simulink model "Falcon"  (R2025b)
settings: Solver=ode1  StartTime=0.0  StopTime=inf  FixedStep=Controller_Sample_Time  RelTol=1e-3  EnableMultiTasking=on
values from neighbouring files (symbols this model uses):
  angles_qcar2 = angles_new_qcar2(2: length (angles_new_qcar2), width (angles_new_qcar2)-5)    [Setup_QCar2_Params.m]
  cal_pos = [0, 0, 0]    [Setup_QCar2_Params.m]
  Controller_Sample_Time = 1/500    (= 0.002)    [Setup_QCar2_Params.m]
  CSI_Sample_Time = Controller_Sample_Time * ceil(0.033 / Controller_Sample_Time)    [Setup_QCar2_Params.m]
  GyroKF_P0 = eye(2)    [Setup_QCar2_Params.m]
  GyroKF_Q = diag([0.01, 0.001])    [Setup_QCar2_Params.m]
  GyroKF_R = 0.01    [Setup_QCar2_Params.m]
  GyroKF_X0 = [0;0]    [Setup_QCar2_Params.m]
  ImageDisplay_Sample_Time = Controller_Sample_Time * 50    (= 0.1)    [Setup_QCar2_Params.m]
  Initialization_Time = 5    [Setup_QCar2_Params.m]
  LiDAR_Sample_Time = Controller_Sample_Time * ceil(1/15 / Controller_Sample_Time)    [Setup_QCar2_Params.m]
  path_x4 = path_x2    [Setup_QCar2_Params.m]
  path_y4 = path_y2    [Setup_QCar2_Params.m]
  qcar2_lidar_to_body_rotation = -pi    (= -3.14159265359)    [Setup_QCar2_Params.m]
  qcar2_lidar_to_map_rotation = 2*pi/180    (= 0.0349065850399)    [Setup_QCar2_Params.m]
  qcar2_virtual_to_physical_lidar_rotation = 0    [Setup_QCar2_Params.m]
  QCarEKF_L = 0.256    [Setup_QCar2_Params.m]
  QCarEKF_P0 = eye(3)    [Setup_QCar2_Params.m]
  QCarEKF_Q = diag([0.00001, 0.00001, 0.00001])    [Setup_QCar2_Params.m]
  QCarEKF_R_combined = diag([0.1, 0.1, 0.01])    [Setup_QCar2_Params.m]
  QCarEKF_R_heading = diag(0.1)    [Setup_QCar2_Params.m]
  QcarKF_X0 = [0; 0; 0]    [Setup_QCar2_Params.m]
  range_qcar2 = distance_new_qcar2(2: length (distance_new_qcar2), width (distance_new_qcar2)-5)    [Setup_QCar2_Params.m]
  RealSense_Sample_Time = Controller_Sample_Time * ceil(0.033 / Controller_Sample_Time)    [Setup_QCar2_Params.m]
  steering_Kd = 0.1    [Setup_QCar2_Params.m]
  steering_Kp = 1    [Setup_QCar2_Params.m]
undefined symbols (not defined in the file or in its folder): AAAF5050, gcbh, height, HIL, JPEG, K12, left, MC, Point, qc_get_step_size, top, video_display_show, width
libraries: quarc_library x45, simulink x3, simulink_extras x3, visionanalysis x1, visiontextngfix x1
(part 3 of 3)

== matlab function Falcon/stateEstimation/Gyro KF + EKF/Heading Kalman Filter ==
  settings: updateMethod=DISCRETE
  data: thd_gyro input; th_gps input; newGPSData input; GyroKF_Q parameter; GyroKF_R parameter; GyroKF_X0 parameter; GyroKF_P0 parameter; th_hat output; gyro_bias output; Controller_Sample_Time parameter
function [th_hat, gyro_bias] = GyroKF(thd_gyro, th_gps, newGPSData, GyroKF_Q, GyroKF_R, GyroKF_X0, GyroKF_P0, Controller_Sample_Time)

    persistent X_hat P I A B C
    if isempty(X_hat)
        % State and Covarience estimates
        X_hat = GyroKF_X0;
        P = GyroKF_P0;

        % Statespace model matrices
        I = eye(2);
        A = I + Controller_Sample_Time*[0, -1;
                                   0, 0];
        B = Controller_Sample_Time*[1;
                               0];
        C = [1, 0];
    end

    % Prediction
    X_hat = A*X_hat + B*thd_gyro;
    P = A*P*A' + GyroKF_Q;

    % Correction 
    if newGPSData
        P_times_CTransposed = P*C';
        S = C*P_times_CTransposed + GyroKF_R;
        K = P_times_CTransposed / S;

        z = wrapToPi(th_gps - C*X_hat);

        X_hat = X_hat + K*z;
        X_hat(1) = wrapToPi(X_hat(1));

        P = (I - K*C) * P;
    end
    
    th_hat = X_hat(1);
    gyro_bias = X_hat(2);
end

== matlab function Falcon/stateEstimation/Gyro KF + EKF/QCar EKF ==
  settings: updateMethod=DISCRETE
  data: speed input; delta input; x_gps input; Xhat output; y_gps input; th_hat input; newGPSData input; Controller_Sample_Time parameter; QCarEKF_P0 parameter; QcarKF_X0 parameter; QCarEKF_R_heading parameter; QCarEKF_Q parameter; QCarEKF_L parameter; QCarEKF_R_combined parameter
function Xhat  = QCarEKF(speed, delta, x_gps, y_gps, th_hat, newGPSData, Controller_Sample_Time, QCarEKF_P0, QcarKF_X0, QCarEKF_R_heading, QCarEKF_Q, QCarEKF_L, QCarEKF_R_combined)




    persistent X_hat P I C_heading C_combined
    if isempty(X_hat)
        % State and Covarience estimates
        X_hat = QcarKF_X0;
        P = QCarEKF_P0;

        % Statespace model matrices
        I = eye(3);
        
        C_heading = [0, 0, 1];
        C_combined = eye(3);
    end
    
    dt = Controller_Sample_Time;
    x = X_hat(1);
    y = X_hat(2);
    th = X_hat(3);
    
    % Prediction:
    F = [1, 0, -dt*speed*sin(th);
         0, 1,  dt*speed*cos(th);
         0, 0,             1];
    P = F*P*F' + QCarEKF_Q;
    
    X_hat = X_hat + dt*speed * [cos(th);
                            sin(th);
                            tan(delta) / QCarEKF_L];
                         
    
    % Correction
    if newGPSData
        y = [x_gps; y_gps; th_hat];
        C = C_combined;
        R = QCarEKF_R_combined;
        
    else
        y = th_hat;
        C = C_heading;
        R = QCarEKF_R_heading;
    end

    P_times_CTransposed = P*C';
    S = C*P_times_CTransposed + R;
    K = P_times_CTransposed / S;

    z = y - C*X_hat;
    if newGPSData
        z(3) = wrapToPi(z(3));
    else
        z = wrapToPi(z);
    end

    X_hat = X_hat + K*z;
    X_hat(3) = wrapToPi(X_hat(3));

    P = (I - K*C) * P;
    
    Xhat = X_hat;
end

== matlab function Falcon/lidarLocalization/Match Scans/MATLAB Function ==
  data: new_range output size=SPR_qcar2 [..SPR_qcar2]; range input [1..SPR_qcar2]; angles input [1..SPR_qcar2]; new_angles output size=SPR_qcar2 [..SPR_qcar2]
function [new_range, new_angles]  = clean_zero_readings(range, angles)
range_indicies = find (range == 0);
range(range_indicies) = [];
angles(range_indicies) = [];
new_range = range;
new_angles = angles;
end

== matlab function Falcon/pathPlanner/Path 4  Look Ahead Generator/Windowed Closest Point Locator *Feedback the location1 ==
  data: x input; location output; y input; x_array input; y_array input; window input; global_search input; distance output; previous_location input
function [location,distance] = find_closest_window_point(x,y,x_array,y_array, window, global_search, previous_location)
distance = 1e6;
location = previous_location;
array_length = length (x_array);

if (global_search == 1)
    
    %Search the whole array (usually at startup)
    for i =1:array_length
        d = (x-x_array(i))^2 + (y-y_array(i))^2;
        if d < distance
            distance = d;
            location = i;
        end
    end
    
else
    
    if (location + window) > array_length
        %We need to wrap from the end
        % loop one - end of array:
        for i = (location-window):array_length
            d = (x-x_array(i))^2 + (y-y_array(i))^2;
            if d < distance
                distance = d;
                location = i;
            end
        end
        % loop two - start of array:
        for i = 1:(location+window-array_length)
            d = (x-x_array(i))^2 + (y-y_array(i))^2;
            if d < distance
                distance = d;
                location = i;
            end
        end
        
    elseif (location-window) < 1
        %We need to wrap from the beginning
        % loop one - end of array:
        for i = (array_length+location-window):array_length
            d = (x-x_array(i))^2 + (y-y_array(i))^2;
            if d < distance
                distance = d;
                location = i;
            end
        end
        % loop two - start of array:
        for i = 1:(location+window)
            d = (x-x_array(i))^2 + (y-y_array(i))^2;
            if d < distance
                distance = d;
                location = i;
            end
        end
        
    else
        %no need to wrap
        for i = (location-window):(location+window)
            d = (x-x_array(i))^2 + (y-y_array(i))^2;
            if d < distance
                distance = d;
                location = i;
            end
        end
    end
    
end
distance = sqrt(distance);
end

== matlab function Falcon/MATLAB Function ==
  data: bboxes input; distance_to_object output; labels input; scores input; depthImg input; object_class output
function [distance_to_object, object_class] = getObjectDepthClass(bboxes, labels, scores, depthImg)

% Default outputs
distance_to_object = single(-1);   % no valid detection / no valid depth
object_class = labels(1);          % placeholder only; ignore when distance_to_object < 0

bestIdx = 0;
bestScore = single(0);

% Pick the detection with the highest positive confidence
for i = 1:size(bboxes,1)
    if isfinite(scores(i)) && ...
       (scores(i) > bestScore) && ...
       (bboxes(i,3) > 1) && ...
       (bboxes(i,4) > 1)

        bestScore = scores(i);
        bestIdx = i;
    end
end

% Only continue if a real detection exists
if bestIdx > 0
    % Return detected class
    object_class = labels(bestIdx);

    % Bounding box = [x y w h]
    x = double(bboxes(bestIdx,1));
    y = double(bboxes(bestIdx,2));
    w = double(bboxes(bestIdx,3));
    h = double(bboxes(bestIdx,4));

    % Depth image size
    H = size(depthImg,1);
    W = size(depthImg,2);

    % Use a small patch around the bbox center
    cx = round(x + w/2);
    cy = round(y + h/2);

    halfW = max(1, round(0.1*w));
    halfH = max(1, round(0.1*h));

    x1 = max(1, cx - halfW);
    x2 = min(W, cx + halfW);
    y1 = max(1, cy - halfH);
    y2 = min(H, cy + halfH);

    % Average valid depth values in the center patch
    sumDepth = single(0);
    count = 0;

    for r = y1:y2
        for c = x1:x2
            d = single(depthImg(r,c));
            if isfinite(d) && (d > 0)
                sumDepth = sumDepth + d;
                count = count + 1;
            end
        end
    end

    % If depth is valid, output it
    if count > 0
        distance_to_object = sumDepth / single(count);

        % Uncomment only if RealSense depth is in millimeters
        % distance_to_object = distance_to_object / 1000;
    else
        % Detection exists but no valid depth in the selected patch
        distance_to_object = single(-1);
    end
end

== matlab function Falcon/PathPlanner ==
  settings: updateMethod=DISCRETE
  data: currentPATHXY input; measuredSpeed input; reset input; Ts input; pickupNode input; dropoffNode input; distance_to_object input; object_class input; targetSpeed output; rgbPct output; leds16 output; rideState output
function [targetSpeed, rgbPct, leds16, rideState] = Main_FSM( ...
    currentPATHXY, measuredSpeed, reset, Ts, pickupNode, dropoffNode, ...
    distance_to_object, object_class)
% =========================================================================
% Perception-Integrated Ride Logic:
%   1) If distance_to_object == -1 -> no perception override
%   2) If distance_to_object <= 1.0 m and STOP SIGN detected:
%         stop for 3.0 s, then continue
%   3) If 1.0 m < distance_to_object <= 1.7 m and RED LIGHT detected:
%         stop and wait until red light disappears
%   4) If GREEN LIGHT detected:
%         no change
%
% NOTE:
%   object_class is assumed to be a numeric/enum class ID.
%   Replace STOP_LABEL_ID, RED_LIGHT_LABEL_ID, GREEN_LIGHT_LABEL_ID below
%   with your actual detector label IDs.
% =========================================================================

% -------------------------
% Detector label IDs (EDIT THESE)
% -------------------------
STOP_LABEL_ID        = int32(3);
RED_LIGHT_LABEL_ID   = int32(2);
GREEN_LIGHT_LABEL_ID = int32(1);

% -------------------------
% Node list (ID -> [x,y])  (26 nodes: 0..25)
% -------------------------
NODE_XY = [ ...
     0.0    ,  0.0   ;  % 0
     0.269  , -0.049 ;  % 1
     1.127  , -1.075 ;  % 2
     1.127  , -0.820 ;  % 3
     2.255  , -0.049 ;  % 4
     1.984  , -0.049 ;  % 5
     1.013  ,  1.081 ;  % 6
     1.235  ,  0.791 ;  % 7
    -0.749  ,  1.077 ;  % 8
    -0.749  ,  0.790 ;  % 9
    -1.282  , -0.59  ;  % 10 (HUB)
     0.0    ,  2.033 ;  % 11
     0.0    ,  1.72  ;  % 12
     0.269  ,  1.72  ;  % 13
     2.255  ,  2.837 ;  % 14
     1.984  ,  1.72  ;  % 15
     0.908  ,  3.58  ;  % 16
     1.466  ,  3.02  ;  % 17
     0.623  ,  2.937 ;  % 18
     0.792  ,  2.729 ;  % 19
     0.0    ,  4.421 ;  % 20
     0.0    ,  4.146 ;  % 21
    -1.984  ,  2.837 ;  % 22
    -1.716  ,  2.837 ;  % 23
    -0.826  ,  3.645 ;  % 24
    -0.857  ,  1.716 ]; % 25

% -------------------------
% Clamp node IDs to valid range [0..25]
% -------------------------
pn = int32(pickupNode);
dn = int32(dropoffNode);
if pn < 0,  pn = int32(0);  end
if pn > 25, pn = int32(25); end
if dn < 0,  dn = int32(0);  end
if dn > 25, dn = int32(25); end

% -------------------------
% Points (meters)
% -------------------------
P0 = NODE_XY(10+1, :).';
P1 = NODE_XY(pn+1,  :).';
P8 = NODE_XY(dn+1,  :).';

% -------------------------
% Parameters
% -------------------------
V_DES_NORMAL      = 0.40;
V_DES_STARTUP     = 0.04;
V_DES_STOPPING    = 0.0;
STARTUP_TIME      = 6.0;

ARRIVE_RADIUS_PICKUP  = 0.30;
ARRIVE_RADIUS_DROPOFF = 0.30;
ARRIVE_RADIUS_HUB     = 0.45;

STOP_SPEED_TH      = 0.05;
STOP_HOLD_TIME     = 3.0;   % standard node stop time
STOP_SIGN_HOLD_SEC = 3.0;   % stop sign hold time

% -------------------------
% Perception distance thresholds
% -------------------------
STOP_SIGN_DIST_MAX = 1;
RED_LIGHT_DIST_MIN = 1;
RED_LIGHT_DIST_MAX = 3;

% -------------------------
% Colors (0..1)
% -------------------------
MAGENTA = [1; 0; 1];
GREEN   = [0; 1; 0];
BLUE    = [0; 0; 1];
ORANGE  = [1; 0.6; 0];
RED     = [1; 0; 0];

% -------------------------
% Car lights
% -------------------------
leds16 = false(16,1);
BRAKES = [11 12 13 14];

% -------------------------
% State machine + timers
% -------------------------
persistent s stopT time arrived1 arrived8 arrived0 spDone lastPick lastDrop
persistent stopSignTimer stopSignActive stopSignServed

if isempty(s) || reset
    s = uint8(0);
    stopT = 0;
    time  = 0;

    stopSignTimer  = 0;
    stopSignActive = false;
    stopSignServed = false;

    arrived1 = false;
    arrived8 = false;
    arrived0 = false;
    spDone = false;
    lastPick = pn;
    lastDrop = dn;
else
    if (pn ~= lastPick) || (dn ~= lastDrop)
        s = uint8(0);
        stopT = 0;
        time  = 0;

        stopSignTimer  = 0;
        stopSignActive = false;
        stopSignServed = false;

        arrived1 = false;
        arrived8 = false;
        arrived0 = false;
        spDone = false;
        lastPick = pn;
        lastDrop = dn;
    end
end

time = time + Ts;

if time < STARTUP_TIME
    V_DES = V_DES_STARTUP;
else
    V_DES = V_DES_NORMAL;
end

% -------------------------
% Current path XY + optional stop flag
% -------------------------
x = currentPATHXY(1);
y = currentPATHXY(2);

stopPoint = false;
if numel(currentPATHXY) >= 3
    stopPoint = (currentPATHXY(3) > 0.5);
end

if ~stopPoint
    spDone = false;
end

d0 = hypot(x - P0(1), y - P0(2));
d1 = hypot(x - P1(1), y - P1(2));
d8 = hypot(x - P8(1), y - P8(2));

% -------------------------
% Stop timer logic
% -------------------------
isStopped = abs(measuredSpeed) < STOP_SPEED_TH;
if isStopped
    stopT = stopT + Ts;
else
    stopT = 0;
end
fullStop = (stopT >= STOP_HOLD_TIME);

% -------------------------
% Drive-state check
% -------------------------
isDriveState = (s==uint8(1)) || (s==uint8(3)) || (s==uint8(5));

% -------------------------
% Perception logic from distance + object class
% -------------------------
validObject = isfinite(distance_to_object) && (distance_to_object >= 0);
objCode = int32(object_class);

isStopSign = validObject && ...
             (distance_to_object <= STOP_SIGN_DIST_MAX) && ...
             (objCode == STOP_LABEL_ID);

isRedLight = validObject && ...
             (distance_to_object > RED_LIGHT_DIST_MIN) && ...
             (distance_to_object <= RED_LIGHT_DIST_MAX) && ...
             (objCode == RED_LIGHT_LABEL_ID);

isGreenLight = validObject && ...
               (objCode == GREEN_LIGHT_LABEL_ID); %#ok<NASGU>

% Re-arm stop sign only after it disappears
if ~isStopSign && ~stopSignActive
    stopSignServed = false;
end

% -------------------------
% Stop-sign override
% Stop 3 seconds, then continue
% Only in drive states
% -------------------------
if isDriveState && isStopSign && ~stopSignActive && ~stopSignServed
    stopSignActive = true;
    stopSignTimer = 0;
end

if stopSignActive
    targetSpeed = V_DES_STOPPING;
    rgbPct = RED;
    leds16(BRAKES) = true;

    stopSignTimer = stopSignTimer + Ts;

    if stopSignTimer >= STOP_SIGN_HOLD_SEC
        stopSignActive = false;
        stopSignServed = true;
        stopSignTimer = 0;
        stopT = 0;
    end

    rideState = double(s);
    return;
end

% -------------------------
% Red-light override
% Stop until red light disappears
% Only in drive states
% -------------------------
if isDriveState && isRedLight
    targetSpeed = V_DES_STOPPING;
    rgbPct = RED;
    leds16(BRAKES) = true;
    rideState = double(s);
    return;
end

% -------------------------
% Green light:
% no change
% -------------------------

% -------------------------
% Stop-Point (Flag-based) Override
% -------------------------
if isDriveState && stopPoint && ~spDone
    targetSpeed = 0;
    rgbPct = RED;
    leds16(BRAKES) = true;

    if fullStop
        spDone = true;
        stopT = 0;
    end

    rideState = double(s);
    return;
end

% -------------------------
% Default Movement
% -------------------------
targetSpeed = V_DES;
rgbPct      = GREEN;

% -------------------------
% Main Mission State Machine
% -------------------------
switch s
    case 0 % HUB_START (Magenta)
        targetSpeed = 0;
        rgbPct = MAGENTA;
        leds16(BRAKES) = true;

        if fullStop
            s = uint8(1);
            stopT = 0;
            arrived1 = false;
            arrived8 = false;
            arrived0 = false;
            spDone = false;
            stopSignActive = false;
            stopSignTimer = 0;
            stopSignServed = false;
        end

    case 1 % DRIVE_TO_PICKUP (Green)
        targetSpeed = V_DES;
        rgbPct = GREEN;

        if d1 < ARRIVE_RADIUS_PICKUP
            arrived1 = true;
        end

        if arrived1
            targetSpeed = 0;
            leds16(BRAKES) = true;
            if fullStop
                s = uint8(2);
                stopT = 0;
            end
        end

    case 2 % PICKUP_STOP (Blue)
        targetSpeed = 0;
        rgbPct = BLUE;
        leds16(BRAKES) = true;

        if fullStop
            s = uint8(3);
            stopT = 0;
        end

    case 3 % DRIVE_TO_DROPOFF (Blue)
        targetSpeed = V_DES;
        rgbPct = BLUE;

        if d8 < ARRIVE_RADIUS_DROPOFF
            arrived8 = true;
        end

        if arrived8
            targetSpeed = 0;
            leds16(BRAKES) = true;
            if fullStop
                s = uint8(4);
                stopT = 0;
            end
        end

    case 4 % DROPOFF_STOP (Orange)
        targetSpeed = 0;
        rgbPct = ORANGE;
        leds16(BRAKES) = true;

        if fullStop
            s = uint8(5);
            stopT = 0;
        end

    case 5 % RETURN_TO_HUB (Orange)
        targetSpeed = V_DES;
        rgbPct = ORANGE;

        if d0 < ARRIVE_RADIUS_HUB
            arrived0 = true;
        end

        if arrived0
            targetSpeed = 0;
            leds16(BRAKES) = true;
            if fullStop
                s = uint8(6);
                stopT = 0;
            end
        end

    case 6 % HUB_END (Magenta)
        targetSpeed = 0;
        rgbPct = MAGENTA;
        leds16(BRAKES) = true;
end

rideState = double(s);
end

% function [targetSpeed, rgbPct, leds16, rideState] = MATLAB_Function( ...
%     currentPATHXY, measuredSpeed, reset, Ts, pickupNode, dropoffNode, visionStop)
% %#codegen
% % =========================================================================
% % Perception-Integrated Ride Logic:
% %   - visionStop: Boolean signal from YOLOX + RealSense Depth logic.
% %   - If visionStop is high during a DRIVE state, car stops for 1.0s.
% % =========================================================================
% 
% % -------------------------
% % Node list (ID -> [x,y])  (26 nodes: 0..25)
% % -------------------------
% NODE_XY = [ ...
%      0.0    ,  0.0   ;  % 0
%      0.269  , -0.049 ;  % 1
%      1.127  , -1.075 ;  % 2
%      1.127  , -0.820 ;  % 3
%      2.255  , -0.049 ;  % 4
%      1.984  , -0.049 ;  % 5
%      1.013  ,  1.081 ;  % 6
%      1.235  ,  0.791 ;  % 7
%     -0.749  ,  1.077 ;  % 8
%     -0.749  ,  0.790 ;  % 9
%     -1.282  , -0.59  ;  % 10 (HUB)
%      0.0    ,  2.033 ;  % 11
%      0.0    ,  1.72  ;  % 12
%      0.269  ,  1.72  ;  % 13
%      2.255  ,  2.837 ;  % 14
%      1.984  ,  1.72  ;  % 15
%      0.908  ,  3.58  ;  % 16
%      1.466  ,  3.02  ;  % 17
%      0.623  ,  2.937 ;  % 18
%      0.792  ,  2.729 ;  % 19
%      0.0    ,  4.421 ;  % 20
%      0.0    ,  4.146 ;  % 21
%     -1.984  ,  2.837 ;  % 22
%     -1.716  ,  2.837 ;  % 23
%     -0.826  ,  3.645 ;  % 24
%     -0.857  ,  1.716 ]; % 25
% 
% % -------------------------
% % Clamp node IDs to valid range [0..25]
% % -------------------------
% pn = int32(pickupNode);
% dn = int32(dropoffNode);
% if pn < 0,  pn = int32(0);  end
% if pn > 25, pn = int32(25); end
% if dn < 0,  dn = int32(0);  end
% if dn > 25, dn = int32(25); end
% 
% % -------------------------
% % Points (meters)
% % -------------------------
% P0 = NODE_XY(10+1, :).';     
% P1 = NODE_XY(pn+1,  :).';    
% P8 = NODE_XY(dn+1,  :).';    
% 
% % -------------------------
% % Parameters
% % -------------------------
% V_DES_NORMAL    = 0.40;   
% V_DES_STARTUP   = 0.04;   
% STARTUP_TIME    = 6.0;    
% 
% ARRIVE_RADIUS_PICKUP  = 0.30;
% ARRIVE_RADIUS_DROPOFF = 0.30;
% ARRIVE_RADIUS_HUB     = 0.45;
% 
% STOP_SPEED_TH   = 0.05;   
% STOP_HOLD_TIME  = 3.0;    % Standard stop time for nodes
% VISION_HOLD_TIME = 1.0;   % Stop time for signs/lights
% 
% % -------------------------
% % Colors (0..1)
% % -------------------------
% MAGENTA = [1; 0; 1];
% GREEN   = [0; 1; 0];
% BLUE    = [0; 0; 1];
% ORANGE  = [1; 0.6; 0];
% RED     = [1; 0; 0];
% 
% % -------------------------
% % Car lights
% % -------------------------
% leds16 = false(16,1);
% BRAKES = [11 12 13 14];
% 
% % -------------------------
% % State machine + timers
% % -------------------------
% persistent s stopT time arrived1 arrived8 arrived0 spDone lastPick lastDrop visionTimer vStopActive
% if isempty(s) || reset
%     s = uint8(0);
%     stopT = 0;
%     time  = 0;
%     visionTimer = 0;
%     vStopActive = false;
%     arrived1 = false;
%     arrived8 = false;
%     arrived0 = false;
%     spDone = false;
%     lastPick = pn;
%     lastDrop = dn;
% else
%     if (pn ~= lastPick) || (dn ~= lastDrop)
%         s = uint8(0);
%         stopT = 0;
%         time  = 0;
%         visionTimer = 0;
%         vStopActive = false;
%         arrived1 = false;
%         arrived8 = false;
%         arrived0 = false;
%         spDone = false;
%         lastPick = pn;
%         lastDrop = dn;
%     end
% end
% 
% time = time + Ts;
% 
% if time < STARTUP_TIME
%     V_DES = V_DES_STARTUP;
% else
%     V_DES = V_DES_NORMAL;
% end
% 
% % -------------------------
% % Current path XY + optional stop flag
% % -------------------------
% x = currentPATHXY(1);
% y = currentPATHXY(2);
% 
% stopPoint = false;
% if (numel(currentPATHXY) >= 3)
%     stopPoint = (currentPATHXY(3) > 0.5);
% end
% 
% if ~stopPoint
%     spDone = false;
% end
% 
% d0 = hypot(x - P0(1), y - P0(2));
% d1 = hypot(x - P1(1), y - P1(2));
% d8 = hypot(x - P8(1), y - P8(2));
% 
% % -------------------------
% % Stop timer logic
% % -------------------------
% isStopped = abs(measuredSpeed) < STOP_SPEED_TH;
% if isStopped
%     stopT = stopT + Ts;
% else
%     stopT = 0;
% end
% fullStop = (stopT >= STOP_HOLD_TIME);
% 
% % -------------------------
% % Perception Override Logic
% % -------------------------
% % Only override during "Drive" states (1, 3, 5)
% isDriveState = (s==uint8(1)) || (s==uint8(3)) || (s==uint8(5));
% 
% if isDriveState && visionStop && ~vStopActive
%     vStopActive = true;
%     visionTimer = 0;
% end
% 
% if vStopActive
%     targetSpeed = 0;
%     rgbPct = RED;
%     leds16(BRAKES) = true;
%     visionTimer = visionTimer + Ts;
% 
%     if visionTimer >= VISION_HOLD_TIME
%         vStopActive = false;
%         visionTimer = 0;
%     end
% 
%     rideState = double(s);
%     return; % Immediate exit to hold stop
% end
% 
% % -------------------------
% % Stop-Point (Flag-based) Override
% % -------------------------
% if isDriveState && stopPoint && ~spDone
%     targetSpeed = 0;
%     rgbPct = RED;
%     leds16(BRAKES) = true;
% 
%     if fullStop
%         spDone = true;   
%         stopT = 0;
%     end
% 
%     rideState = double(s);
%     return;
% end
% 
% % -------------------------
% % Default Movement
% % -------------------------
% targetSpeed = V_DES;
% rgbPct      = GREEN;
% 
% % -------------------------
% % Main Mission State Machine
% % -------------------------
% switch s
%     case 0 % HUB_START (Magenta)
%         targetSpeed = 0;
%         rgbPct = MAGENTA;
%         leds16(BRAKES) = true;
%         if fullStop
%             s = uint8(1);
%             stopT = 0;
%             arrived1 = false; arrived8 = false; arrived0 = false; spDone = false;
%         end
% 
%     case 1 % DRIVE_TO_PICKUP (Green)
%         targetSpeed = V_DES;
%         rgbPct = GREEN;
%         if d1 < ARRIVE_RADIUS_PICKUP, arrived1 = true; end
%         if arrived1
%             targetSpeed = 0;
%             leds16(BRAKES) = true;
%             if fullStop
%                 s = uint8(2);
%                 stopT = 0;
%             end
%         end
% 
%     case 2 % PICKUP_STOP (Blue)
%         targetSpeed = 0;
%         rgbPct = BLUE;
%         leds16(BRAKES) = true;
%         if fullStop
%             s = uint8(3);
%             stopT = 0;
%         end
% 
%     case 3 % DRIVE_TO_DROPOFF (Blue)
%         targetSpeed = V_DES;
%         rgbPct = BLUE;
%         if d8 < ARRIVE_RADIUS_DROPOFF, arrived8 = true; end
%         if arrived8
%             targetSpeed = 0;
%             leds16(BRAKES) = true;
%             if fullStop
%                 s = uint8(4);
%                 stopT = 0;
%             end
%         end
% 
%     case 4 % DROPOFF_STOP (Orange)
%         targetSpeed = 0;
%         rgbPct = ORANGE;
%         leds16(BRAKES) = true;
%         if fullStop
%             s = uint8(5);
%             stopT = 0;
%         end
% 
%     case 5 % RETURN_TO_HUB (Orange)
%         targetSpeed = V_DES;
%         rgbPct = ORANGE;
%         if d0 < ARRIVE_RADIUS_HUB, arrived0 = true; end
%         if arrived0
%             targetSpeed = 0;
%             leds16(BRAKES) = true;
%             if fullStop
%                 s = uint8(6);
%                 stopT = 0;
%             end
%         end
% 
%     case 6 % HUB_END (Magenta)
%         targetSpeed = 0;
%         rgbPct = MAGENTA;
%         leds16(BRAKES) = true;
% end
% 
% rideState = double(s);
% end

== matlab function Falcon/stateEstimation/Sensor Fusion - Complementary Filter/MATLAB Function ==
  data: car_speed input; correction_weight output; slope input; min_weight input
function correction_weight = weighting(car_speed, slope, min_weight)
correction_weight = 1 - 1*slope*car_speed;
if correction_weight < min_weight
    correction_weight = min_weight;
end
end

== matlab function Falcon/speedController/realsenseObstacleDetectionSpeedAdjust/MATLAB Function ==
  data: obstacle_distance input; speed_cmd output; stop_distance input; nominal_tracking_distance input; nominal_speed input
function speed_cmd = adaptive_cruise_control(obstacle_distance, stop_distance, nominal_tracking_distance, nominal_speed)

speed_cmd = nominal_speed;

if obstacle_distance < stop_distance
    speed_cmd = sat(nominal_speed,0,-1);
    
elseif obstacle_distance < nominal_tracking_distance
    speed_cmd = nominal_speed/(nominal_tracking_distance-stop_distance)*obstacle_distance...
        - nominal_speed/(nominal_tracking_distance-stop_distance)*stop_distance;
    
end

function output = sat (input, max,min)
if input > max
    output = max;
elseif input < min
    output = min;
else
    output = input;
end
